simulink library "Lib_Decoder"  (R2012b)
settings: Solver=ode45  StartTime=0.0  StopTime=10.0  RelTol=1e-3
settings Model: Creator=gilja  LastModifiedBy=NPTL

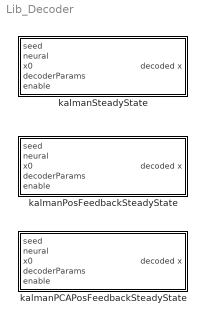
== system Lib_Decoder ==
  kalmanPCAPosFeedbackSteadyState : Subsystem
  kalmanPosFeedbackSteadyState : Subsystem
  kalmanSteadyState : Subsystem

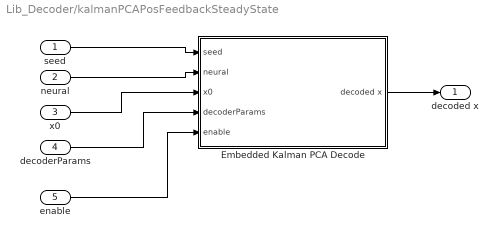
== system Lib_Decoder/kalmanPCAPosFeedbackSteadyState ==
  seed : Inport
  neural : Inport  Port=2
  x0 : Inport  Port=3
  decoderParams : Inport  Port=4
  enable : Inport  Port=5
  Embedded Kalman PCA Decode : Subsystem
  decoded x : Outport
  wires:
  Embedded Kalman PCA Decode/1(decoded x) -> decoded x/1
  seed/1 -> Embedded Kalman PCA Decode/1(seed)
  neural/1 -> Embedded Kalman PCA Decode/2(neural)
  x0/1 -> Embedded Kalman PCA Decode/3(x0)
  decoderParams/1 -> Embedded Kalman PCA Decode/4(decoderParams)
  enable/1 -> Embedded Kalman PCA Decode/5(enable)

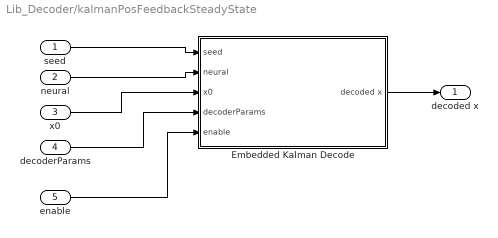
== system Lib_Decoder/kalmanPosFeedbackSteadyState ==
  seed : Inport
  neural : Inport  Port=2
  x0 : Inport  Port=3
  decoderParams : Inport  Port=4
  enable : Inport  Port=5
  Embedded Kalman Decode : Subsystem
  decoded x : Outport
  wires:
  Embedded Kalman Decode/1(decoded x) -> decoded x/1
  seed/1 -> Embedded Kalman Decode/1(seed)
  neural/1 -> Embedded Kalman Decode/2(neural)
  x0/1 -> Embedded Kalman Decode/3(x0)
  decoderParams/1 -> Embedded Kalman Decode/4(decoderParams)
  enable/1 -> Embedded Kalman Decode/5(enable)

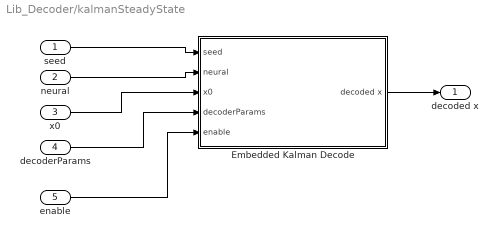
== system Lib_Decoder/kalmanSteadyState ==
  seed : Inport
  neural : Inport  Port=2
  x0 : Inport  Port=3
  decoderParams : Inport  Port=4
  enable : Inport  Port=5
  Embedded Kalman Decode : Subsystem
  decoded x : Outport
  wires:
  Embedded Kalman Decode/1(decoded x) -> decoded x/1
  seed/1 -> Embedded Kalman Decode/1(seed)
  neural/1 -> Embedded Kalman Decode/2(neural)
  x0/1 -> Embedded Kalman Decode/3(x0)
  decoderParams/1 -> Embedded Kalman Decode/4(decoderParams)
  enable/1 -> Embedded Kalman Decode/5(enable)

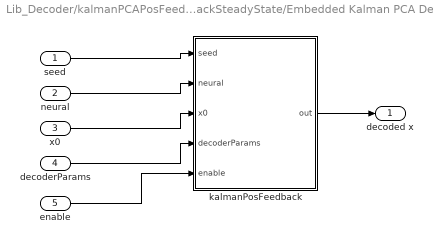
== system Lib_Decoder/kalmanPCAPosFeedbackSteadyState/Embedded Kalman PCA Decode ==
  seed : Inport
  neural : Inport  Port=2
  x0 : Inport  Port=3
  decoderParams : Inport  Port=4
  enable : Inport  Port=5
  kalmanPosFeedback : MATLAB Function  TreatAsAtomicUnit=on
  decoded x : Outport
  wires:
  kalmanPosFeedback/1(out) -> decoded x/1
  seed/1 -> kalmanPosFeedback/1(seed)
  neural/1 -> kalmanPosFeedback/2(neural)
  x0/1 -> kalmanPosFeedback/3(x0)
  decoderParams/1 -> kalmanPosFeedback/4(decoderParams)
  enable/1 -> kalmanPosFeedback/5(enable)

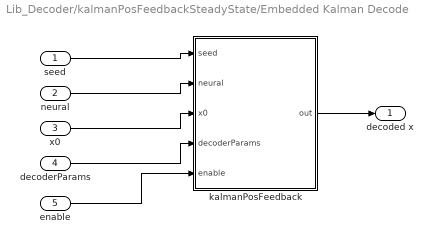
== system Lib_Decoder/kalmanPosFeedbackSteadyState/Embedded Kalman Decode ==
  seed : Inport
  neural : Inport  Port=2
  x0 : Inport  Port=3
  decoderParams : Inport  Port=4
  enable : Inport  Port=5
  kalmanPosFeedback : MATLAB Function  TreatAsAtomicUnit=on
  decoded x : Outport
  wires:
  kalmanPosFeedback/1(out) -> decoded x/1
  seed/1 -> kalmanPosFeedback/1(seed)
  neural/1 -> kalmanPosFeedback/2(neural)
  x0/1 -> kalmanPosFeedback/3(x0)
  decoderParams/1 -> kalmanPosFeedback/4(decoderParams)
  enable/1 -> kalmanPosFeedback/5(enable)

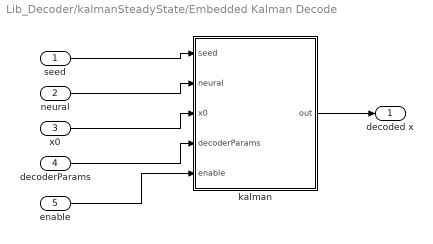
== system Lib_Decoder/kalmanSteadyState/Embedded Kalman Decode ==
  seed : Inport
  neural : Inport  Port=2
  x0 : Inport  Port=3
  decoderParams : Inport  Port=4
  enable : Inport  Port=5
  kalman : MATLAB Function  TreatAsAtomicUnit=on
  decoded x : Outport
  wires:
  kalman/1(out) -> decoded x/1
  seed/1 -> kalman/1(seed)
  neural/1 -> kalman/2(neural)
  x0/1 -> kalman/3(x0)
  decoderParams/1 -> kalman/4(decoderParams)
  enable/1 -> kalman/5(enable)

== matlab function Lib_Decoder/kalmanPosFeedbackSteadyState/Embedded Kalman Decode/kalmanPosFeedback ==
  data: seed input; neural input; x0 input; out output; decoderParams input; enable input
function out = kalmanPosFeedback(seed, neural, x0, decoderParams, enable)
%% steady state kalman filter

%     persistent A C K;
persistent xout;

A = decoderParams.A;
C = decoderParams.C;
Cfeedback = decoderParams.Cfeedback;
K = decoderParams.K;
transform = decoderParams.transform;

if isempty(xout)
    xout = x0;
    xout(end) = 1;
end

if seed
    xout = x0;
elseif enable
    xkprior = A*x0;
    switch transform
        case DecoderConstants.NO_TRANSFORM
            xout = xkprior + K*(neural(:)-Cfeedback*xkprior - C*xkprior);
        case DecoderTransforms.SQRT_TRANSFORM
            xout = xkprior + K*(sqrt(neural(:))-Cfeedback*xkprior - C*xkprior);
    end
end

out = xout;
end

== matlab function Lib_Decoder/kalmanPCAPosFeedbackSteadyState/Embedded Kalman PCA Decode/kalmanPosFeedback ==
  data: seed input; neural input; x0 input; out output; decoderParams input; enable input
function out = kalmanPosFeedback(seed, neural, x0, decoderParams, enable)
%% steady state kalman filter

%     persistent A C K;
persistent xout;

A = decoderParams.A;
C = decoderParams.C;
Cfeedback = decoderParams.Cfeedback;
K = decoderParams.K;
transform = decoderParams.transform;
decoderType = decoderParams.decoderType;
projector = decoderParams.projector;
invSoftNormVals = decoderParams.invSoftNormVals;
pcaMeans = decoderParams.pcaMeans;
pcaDims = decoderParams.pcaDims;

projN = zeros(size(neural(:)));

if isempty(xout)
    xout = x0;
    xout(end) = 1;
    
end

if seed
    xout = x0;
elseif enable
    switch decoderType
        case DecoderConstants.DECODER_TYPE_VFBSSKF
            xkprior = A*x0;
            switch transform
                case DecoderConstants.NO_TRANSFORM
                    xout = xkprior + K*(neural(:)-Cfeedback*xkprior - C*xkprior);
                case DecoderConstants.SQRT_TRANSFORM
                    xout = xkprior + K*(sqrt(neural(:))-Cfeedback*xkprior - C*xkprior);
            end
        case DecoderConstants.DECODER_TYPE_PCAVFBSSKF
            if (any(invSoftNormVals))
                neural(:) = neural(:) .* invSoftNormVals;
            end
            
            neural(:) = neural(:) - pcaMeans;
            
            projN = projector' * neural(:);
            
            xkprior = A*x0;
            xout = xkprior + K*(projN-Cfeedback*xkprior - C*xkprior);
    end
end
out = xout;
end

== matlab function Lib_Decoder/kalmanSteadyState/Embedded Kalman Decode/kalman ==
  data: seed input; neural input; x0 input; out output; decoderParams input; enable input
function out = kalman(seed, neural, x0, decoderParams, enable)
%% steady state kalman filter

%     persistent A C K;
persistent xout;

A = decoderParams.A;
C = decoderParams.C;
K = decoderParams.K;

if isempty(xout)
    xout = x0;
    xout(end) = 1;
end

if seed
    xout = x0;
elseif enable
    xkprior = A*x0;
    xout = xkprior + K*(neural(:) - C*xkprior);
end

out = xout;
end
